simulink model "ltao_v1"  (R2022b)
settings: Solver=FixedStepDiscrete  StartTime=0.0  StopTime=0.6  FixedStep=FEM_Ts  MaxStep=FEM_Ts  RelTol=1e-2
InitFcn:
  | %
  | % Initialization callback function
  | %
  | 
  | try
  |    fprintf('\nGMT IMS version (%s)!\n',simulink_fname );
  | 
  |    % Get Simulink model directory
  |    [filepath,name,ext] = fileparts(which(bdroot));
  | 
  |    if ~strcmp(filepath,pwd)
  |       fprintf('\nChanging current directory to \n %s \n',filepath);
  |       cd(filepath);
  |    end
  | 
  |    %
  |  if(osim.bpless_wl)
  |     fprintf('Generating bumpless wind load time series\n');
  |  end
  | catch
  |    warning('Running the InitFcn from puSimulate script');
  | end
values from neighbouring files (symbols this model uses):
  asm_ssG = XiKL' * asm_ssG * XiKL    [load_ltao_e2e.m]
  Cpi_d = eye(n_Zmodes)* c2d(st.asm.fpi, Ts, c2d_opts)    [evalM2asm_modal.m]    (also in load_ltao_e2e.m = c2d(st.asm.fpi, FEM_Ts, c2d_opts))
  fao_d = c2d(st.glao.fao, st.glao.T, c2d_opts)    [evalM2asm_modal.m]    (also in load_ltao_e2e.m = c2d(st.ltao.fao, FEM_Ts, c2d_opts))
  fao_d4k = c2d(st.ltao.fao, 1/4e3, c2d_opts)    [evalM2asm_modal.m]    (also in load_ltao_e2e.m = c2d(st.ltao.fao, FEM_Ts, c2d_opts))
  FEM_Ts = 1/8e3    (= 0.000125)    [load_ltao_e2e.m]
  fes = c2d(tf((fc_es^2)*4*(pi^2),[1, 2*0.8*fc_es*2*pi, (fc_es^2)*4*(pi^2)]),     st.ltao.T,c2d_opts)    [load_ltao_e2e.m]
  flag_1stOdyn_d = tf(c2d(flag(2,1), Ts, c2d_opts))    [evalM2asm_modal.m]    (also in load_ltao_e2e.m = tf(c2d(flag(2,1),FEM_Ts,c2d_opts)))
  flag_2ndOdyn_d = tf(c2d(flag(3,1), Ts, c2d_opts))    [evalM2asm_modal.m]    (also in load_ltao_e2e.m = tf(c2d(flag(3,1),FEM_Ts,c2d_opts)))
  fpre_d = tf(c2d(st.asm.fpre, Ts, c2d_opts))    [evalM2asm_modal.m]    (also in load_ltao_e2e.m = tf(c2d(fpre,FEM_Ts,c2d_opts)))
  gtt2mnt = eye(2)/(rbm2gtt * Hk_mnt_m1m2)    [load_ltao_e2e.m]
  Hk_mnt_m1m2 = Cm1m2*pinv(Cmnt)    [load_ltao_e2e.m]
  Hpd_d = eye(n_Zmodes)* c2d(st.asm.fpd, Ts, c2d_opts)    [evalM2asm_modal.m]    (also in load_ltao_e2e.m = c2d(st.asm.fpd, FEM_Ts, 'Tustin'))
  Km1rbm_es = (KhpF2es/KhpF2m1rbm)    [load_ltao_e2e.m]
  Ks = cell(7,1)    [load_ltao_e2e.m]
  m1m2_segP_dist = [zeros(42,1); 1e-5*randn(42,1)]    [load_ltao_e2e.m]
  PG = zeros(length(om2),6)    [evalM2asm_modal.m]    (also in load_ltao_e2e.m)
  phiB = inputs2ModalF(mode_ind_vec,indDesInputs) * KinputT    [load_ltao_e2e.m]
  phiC = KoutputT * modalDisp2Outputs(indDesOutputs,mode_ind_vec)    [load_ltao_e2e.m]
  Psi_ss = KoutputT *gainMatrix(indDesOutputs,indDesInputs)* KinputT - K_ss    [load_ltao_e2e.m]
  segPTT2asmCMD = cell(7,1)    [load_ltao_e2e.m]
  Sm1m2_gtt = (Hk_mnt_m1m2*gtt2mnt) * rbm2gtt    [load_ltao_e2e.m]
  st = getcontrol_asm()    [evalM2asm_modal.m]    (also in load_ltao_e2e.m)
undefined symbols (not defined in the file or in its folder): a, az, az_ff_en, b, c, D_seg_piston, D_seg_tt, DiscIntNeverNeededParam, el, fem, gir, m1sys, m2_rbm_dist, m2pos, magnitude, mount, osim, rbm2gtt, Rm1es, Rm2es, sm, VC_modal_stiff
libraries: ims_block_library x7, simulink x2
(part 2 of 3)

== system ltao_v1/ASMmodal_Control/ASM_inner_loop_controller_S1 ==
  ASM_cmd : Inport
  ASM_FB : Inport  Port=2
  ASM Input filter : DiscreteTransferFcn  Numerator=fpre_d.num{1}  Denominator=fpre_d.den{1}  SampleTime=fpre_d.Ts
  ASM PI controller : DiscreteTransferFcn  Numerator=Cpi_d.num{1}  Denominator=Cpi_d.den{1}  SampleTime=Cpi_d.Ts
  Kb : Gain  Gain=st.asm.Kb
  Kd : Gain  Gain=st.asm.Kd
  Km : Gain  Gain=st.asm.Km
  Ks : Gain  Gain=Ks{1}  Multiplication=Matrix(K*u)
  Numerical differentiation : DiscreteTransferFcn  Numerator=Hpd_d.num{1}  Denominator=Hpd_d.den{1}  SampleTime=Hpd_d.Ts
  Sum1 : Sum  Inputs=|+-
  Sum2 : Sum
  Sum3 : Sum  Inputs=|+-
  Sum4 : Sum  Inputs=++|
  Sum5 : Sum
  m2_asm_ff_en : Gain  Gain=osim.m2_asm_ff_en
  s*fpre (DT version) : DiscreteTransferFcn  Numerator=flag_1stOdyn_d.num{1}  Denominator=flag_1stOdyn_d.den{1}  SampleTime=flag_1stOdyn_d.Ts
  s^2*fpre (DT version) : DiscreteTransferFcn  Numerator=flag_2ndOdyn_d.num{1}  Denominator=flag_2ndOdyn_d.den{1}  SampleTime=flag_2ndOdyn_d.Ts
  ASM_modalF : Outport  VectorParamsAs1DForOutWhenUnconnected=off
  Mag_modal_vel : Outport  Port=2  VectorParamsAs1DForOutWhenUnconnected=off
  wires:
  m2_asm_ff_en/1 -> Sum4/1
  s*fpre (DT version)/1 -> Kb/1
  ASM PI controller/1 -> Sum3/1
  Sum3/1 -> Sum4/2
  Km/1 -> Sum5/1
  Kb/1 -> Sum5/2
  Ks/1 -> Sum2/2
  s^2*fpre (DT version)/1 -> Km/1
  Kd/1 -> Sum3/2
  Sum5/1 -> Sum2/1
  ASM_FB/1 -> Numerical differentiation/1, Sum1/2
  ASM_cmd/1 -> s^2*fpre (DT version)/1, s*fpre (DT version)/1, ASM Input filter/1
  Sum1/1 -> ASM PI controller/1
  Sum4/1 -> ASM_modalF/1
  Sum2/1 -> m2_asm_ff_en/1
  Numerical differentiation/1 -> Mag_modal_vel/1, Kd/1
  ASM Input filter/1 -> Ks/1, Sum1/1

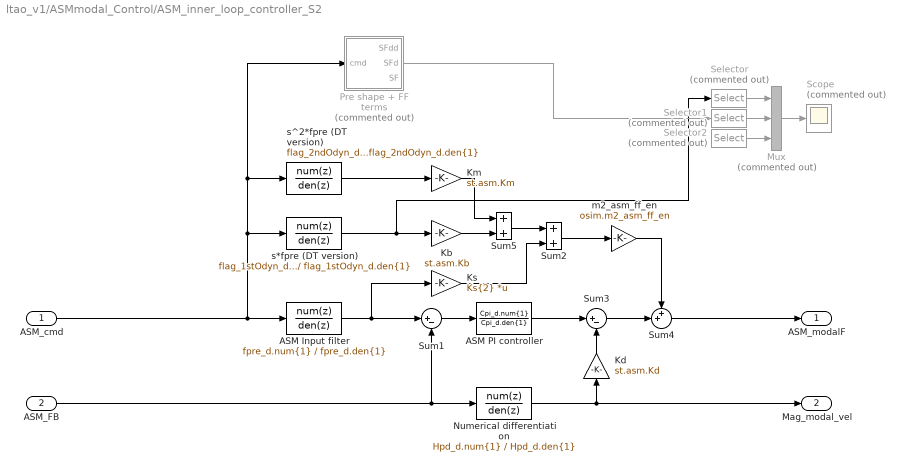
== system ltao_v1/ASMmodal_Control/ASM_inner_loop_controller_S2 ==
  ASM_cmd : Inport
  ASM_FB : Inport  Port=2
  ASM Input filter : DiscreteTransferFcn  Numerator=fpre_d.num{1}  Denominator=fpre_d.den{1}  SampleTime=fpre_d.Ts
  ASM PI controller : DiscreteTransferFcn  Numerator=Cpi_d.num{1}  Denominator=Cpi_d.den{1}  SampleTime=Cpi_d.Ts
  Kb : Gain  Gain=st.asm.Kb
  Kd : Gain  Gain=st.asm.Kd
  Km : Gain  Gain=st.asm.Km
  Ks : Gain  Gain=Ks{2}  Multiplication=Matrix(K*u)
  Mux : Mux  Commented=on  Inputs=3
  Numerical differentiation : DiscreteTransferFcn  Numerator=Hpd_d.num{1}  Denominator=Hpd_d.den{1}  SampleTime=Hpd_d.Ts
  Pre shape + FF terms : Subsystem  Commented=on
  Scope : Scope  Commented=on
  Selector : Selector  Commented=on  InputPortWidth=66  IndexOptions=Index vector (dialog)  Indices=[1 4]  OutputSizes=1
  Selector1 : Selector  Commented=on  InputPortWidth=66  IndexOptions=Index vector (dialog)  Indices=[1 4]  OutputSizes=1
  Selector2 : Selector  Commented=on  InputPortWidth=66  IndexOptions=Index vector (dialog)  Indices=[1 4]  OutputSizes=1
  Sum1 : Sum  Inputs=|+-
  Sum2 : Sum
  Sum3 : Sum  Inputs=|+-
  Sum4 : Sum  Inputs=++|
  Sum5 : Sum
  m2_asm_ff_en : Gain  Gain=osim.m2_asm_ff_en
  s*fpre (DT version) : DiscreteTransferFcn  Numerator=flag_1stOdyn_d.num{1}  Denominator=flag_1stOdyn_d.den{1}  SampleTime=flag_1stOdyn_d.Ts
  s^2*fpre (DT version) : DiscreteTransferFcn  Numerator=flag_2ndOdyn_d.num{1}  Denominator=flag_2ndOdyn_d.den{1}  SampleTime=flag_2ndOdyn_d.Ts
  ASM_modalF : Outport  VectorParamsAs1DForOutWhenUnconnected=off
  Mag_modal_vel : Outport  Port=2  VectorParamsAs1DForOutWhenUnconnected=off
  wires:
  s*fpre (DT version)/1 -> Selector/1, Kb/1
  ASM PI controller/1 -> Sum3/1
  Sum3/1 -> Sum4/2
  Km/1 -> Sum5/1
  Kb/1 -> Sum5/2
  Ks/1 -> Sum2/2
  s^2*fpre (DT version)/1 -> Km/1
  Kd/1 -> Sum3/2
  Sum5/1 -> Sum2/1
  ASM_FB/1 -> Numerical differentiation/1, Sum1/2
  ASM_cmd/1 -> Pre shape + FF terms/1(cmd), s^2*fpre (DT version)/1, s*fpre (DT version)/1, ASM Input filter/1
  Sum1/1 -> ASM PI controller/1
  Sum4/1 -> ASM_modalF/1
  Sum2/1 -> m2_asm_ff_en/1
  Numerical differentiation/1 -> Mag_modal_vel/1, Kd/1
  ASM Input filter/1 -> Ks/1, Sum1/1
  Mux/1 -> Scope/1
  Selector1/1 -> Mux/2
  Selector/1 -> Mux/1
  Selector2/1 -> Mux/3
  m2_asm_ff_en/1 -> Sum4/1
  Pre shape + FF terms/2(SFd) -> Selector1/1

== system ltao_v1/ASMmodal_Control/ASM_inner_loop_controller_S3 ==
  ASM_cmd : Inport
  ASM_FB : Inport  Port=2
  ASM Input filter : DiscreteTransferFcn  Numerator=fpre_d.num{1}  Denominator=fpre_d.den{1}  SampleTime=fpre_d.Ts
  ASM PI controller : DiscreteTransferFcn  Numerator=Cpi_d.num{1}  Denominator=Cpi_d.den{1}  SampleTime=Cpi_d.Ts
  Kb : Gain  Gain=st.asm.Kb
  Kd : Gain  Gain=st.asm.Kd
  Km : Gain  Gain=st.asm.Km
  Ks : Gain  Gain=Ks{3}  Multiplication=Matrix(K*u)
  Numerical differentiation : DiscreteTransferFcn  Numerator=Hpd_d.num{1}  Denominator=Hpd_d.den{1}  SampleTime=Hpd_d.Ts
  Sum1 : Sum  Inputs=|+-
  Sum2 : Sum
  Sum3 : Sum  Inputs=|+-
  Sum4 : Sum  Inputs=++|
  Sum5 : Sum
  m2_asm_ff_en : Gain  Gain=osim.m2_asm_ff_en
  s*fpre (DT version) : DiscreteTransferFcn  Numerator=flag_1stOdyn_d.num{1}  Denominator=flag_1stOdyn_d.den{1}  SampleTime=flag_1stOdyn_d.Ts
  s^2*fpre (DT version) : DiscreteTransferFcn  Numerator=flag_2ndOdyn_d.num{1}  Denominator=flag_2ndOdyn_d.den{1}  SampleTime=flag_2ndOdyn_d.Ts
  ASM_modalF : Outport  VectorParamsAs1DForOutWhenUnconnected=off
  Mag_modal_vel : Outport  Port=2  VectorParamsAs1DForOutWhenUnconnected=off
  wires:
  m2_asm_ff_en/1 -> Sum4/1
  s*fpre (DT version)/1 -> Kb/1
  ASM PI controller/1 -> Sum3/1
  Sum3/1 -> Sum4/2
  Km/1 -> Sum5/1
  Kb/1 -> Sum5/2
  Ks/1 -> Sum2/2
  s^2*fpre (DT version)/1 -> Km/1
  Kd/1 -> Sum3/2
  Sum5/1 -> Sum2/1
  ASM_FB/1 -> Numerical differentiation/1, Sum1/2
  ASM_cmd/1 -> s^2*fpre (DT version)/1, s*fpre (DT version)/1, ASM Input filter/1
  Sum1/1 -> ASM PI controller/1
  Sum4/1 -> ASM_modalF/1
  Sum2/1 -> m2_asm_ff_en/1
  Numerical differentiation/1 -> Mag_modal_vel/1, Kd/1
  ASM Input filter/1 -> Ks/1, Sum1/1

== system ltao_v1/ASMmodal_Control/ASM_inner_loop_controller_S4 ==
  ASM_cmd : Inport
  ASM_FB : Inport  Port=2
  ASM Input filter : DiscreteTransferFcn  Numerator=fpre_d.num{1}  Denominator=fpre_d.den{1}  SampleTime=fpre_d.Ts
  ASM PI controller : DiscreteTransferFcn  Numerator=Cpi_d.num{1}  Denominator=Cpi_d.den{1}  SampleTime=Cpi_d.Ts
  Kb : Gain  Gain=st.asm.Kb
  Kd : Gain  Gain=st.asm.Kd
  Km : Gain  Gain=st.asm.Km
  Ks : Gain  Gain=Ks{4}  Multiplication=Matrix(K*u)
  Numerical differentiation : DiscreteTransferFcn  Numerator=Hpd_d.num{1}  Denominator=Hpd_d.den{1}  SampleTime=Hpd_d.Ts
  Sum1 : Sum  Inputs=|+-
  Sum2 : Sum
  Sum3 : Sum  Inputs=|+-
  Sum4 : Sum  Inputs=++|
  Sum5 : Sum
  m2_asm_ff_en : Gain  Gain=osim.m2_asm_ff_en
  s*fpre (DT version) : DiscreteTransferFcn  Numerator=flag_1stOdyn_d.num{1}  Denominator=flag_1stOdyn_d.den{1}  SampleTime=flag_1stOdyn_d.Ts
  s^2*fpre (DT version) : DiscreteTransferFcn  Numerator=flag_2ndOdyn_d.num{1}  Denominator=flag_2ndOdyn_d.den{1}  SampleTime=flag_2ndOdyn_d.Ts
  ASM_modalF : Outport  VectorParamsAs1DForOutWhenUnconnected=off
  Mag_modal_vel : Outport  Port=2  VectorParamsAs1DForOutWhenUnconnected=off
  wires:
  m2_asm_ff_en/1 -> Sum4/1
  s*fpre (DT version)/1 -> Kb/1
  ASM PI controller/1 -> Sum3/1
  Sum3/1 -> Sum4/2
  Km/1 -> Sum5/1
  Kb/1 -> Sum5/2
  Ks/1 -> Sum2/2
  s^2*fpre (DT version)/1 -> Km/1
  Kd/1 -> Sum3/2
  Sum5/1 -> Sum2/1
  ASM_FB/1 -> Numerical differentiation/1, Sum1/2
  ASM_cmd/1 -> s^2*fpre (DT version)/1, s*fpre (DT version)/1, ASM Input filter/1
  Sum1/1 -> ASM PI controller/1
  Sum4/1 -> ASM_modalF/1
  Sum2/1 -> m2_asm_ff_en/1
  Numerical differentiation/1 -> Mag_modal_vel/1, Kd/1
  ASM Input filter/1 -> Ks/1, Sum1/1

== system ltao_v1/ASMmodal_Control/ASM_inner_loop_controller_S5 ==
  ASM_cmd : Inport
  ASM_FB : Inport  Port=2
  ASM Input filter : DiscreteTransferFcn  Numerator=fpre_d.num{1}  Denominator=fpre_d.den{1}  SampleTime=fpre_d.Ts
  ASM PI controller : DiscreteTransferFcn  Numerator=Cpi_d.num{1}  Denominator=Cpi_d.den{1}  SampleTime=Cpi_d.Ts
  Kb : Gain  Gain=st.asm.Kb
  Kd : Gain  Gain=st.asm.Kd
  Km : Gain  Gain=st.asm.Km
  Ks : Gain  Gain=Ks{5}  Multiplication=Matrix(K*u)
  Numerical differentiation : DiscreteTransferFcn  Numerator=Hpd_d.num{1}  Denominator=Hpd_d.den{1}  SampleTime=Hpd_d.Ts
  Sum1 : Sum  Inputs=|+-
  Sum2 : Sum
  Sum3 : Sum  Inputs=|+-
  Sum4 : Sum  Inputs=++|
  Sum5 : Sum
  m2_asm_ff_en : Gain  Gain=osim.m2_asm_ff_en
  s*fpre (DT version) : DiscreteTransferFcn  Numerator=flag_1stOdyn_d.num{1}  Denominator=flag_1stOdyn_d.den{1}  SampleTime=flag_1stOdyn_d.Ts
  s^2*fpre (DT version) : DiscreteTransferFcn  Numerator=flag_2ndOdyn_d.num{1}  Denominator=flag_2ndOdyn_d.den{1}  SampleTime=flag_2ndOdyn_d.Ts
  ASM_modalF : Outport  VectorParamsAs1DForOutWhenUnconnected=off
  Mag_modal_vel : Outport  Port=2  VectorParamsAs1DForOutWhenUnconnected=off
  wires:
  m2_asm_ff_en/1 -> Sum4/1
  s*fpre (DT version)/1 -> Kb/1
  ASM PI controller/1 -> Sum3/1
  Sum3/1 -> Sum4/2
  Km/1 -> Sum5/1
  Kb/1 -> Sum5/2
  Ks/1 -> Sum2/2
  s^2*fpre (DT version)/1 -> Km/1
  Kd/1 -> Sum3/2
  Sum5/1 -> Sum2/1
  ASM_FB/1 -> Numerical differentiation/1, Sum1/2
  ASM_cmd/1 -> s^2*fpre (DT version)/1, s*fpre (DT version)/1, ASM Input filter/1
  Sum1/1 -> ASM PI controller/1
  Sum4/1 -> ASM_modalF/1
  Sum2/1 -> m2_asm_ff_en/1
  Numerical differentiation/1 -> Mag_modal_vel/1, Kd/1
  ASM Input filter/1 -> Ks/1, Sum1/1

== system ltao_v1/ASMmodal_Control/ASM_inner_loop_controller_S6 ==
  ASM_cmd : Inport
  ASM_FB : Inport  Port=2
  ASM Input filter : DiscreteTransferFcn  Numerator=fpre_d.num{1}  Denominator=fpre_d.den{1}  SampleTime=fpre_d.Ts
  ASM PI controller : DiscreteTransferFcn  Numerator=Cpi_d.num{1}  Denominator=Cpi_d.den{1}  SampleTime=Cpi_d.Ts
  Kb : Gain  Gain=st.asm.Kb
  Kd : Gain  Gain=st.asm.Kd
  Km : Gain  Gain=st.asm.Km
  Ks : Gain  Gain=Ks{6}  Multiplication=Matrix(K*u)
  Numerical differentiation : DiscreteTransferFcn  Numerator=Hpd_d.num{1}  Denominator=Hpd_d.den{1}  SampleTime=Hpd_d.Ts
  Sum1 : Sum  Inputs=|+-
  Sum2 : Sum
  Sum3 : Sum  Inputs=|+-
  Sum4 : Sum  Inputs=++|
  Sum5 : Sum
  m2_asm_ff_en : Gain  Gain=osim.m2_asm_ff_en
  s*fpre (DT version) : DiscreteTransferFcn  Numerator=flag_1stOdyn_d.num{1}  Denominator=flag_1stOdyn_d.den{1}  SampleTime=flag_1stOdyn_d.Ts
  s^2*fpre (DT version) : DiscreteTransferFcn  Numerator=flag_2ndOdyn_d.num{1}  Denominator=flag_2ndOdyn_d.den{1}  SampleTime=flag_2ndOdyn_d.Ts
  ASM_modalF : Outport  VectorParamsAs1DForOutWhenUnconnected=off
  Mag_modal_vel : Outport  Port=2  VectorParamsAs1DForOutWhenUnconnected=off
  wires:
  m2_asm_ff_en/1 -> Sum4/1
  s*fpre (DT version)/1 -> Kb/1
  ASM PI controller/1 -> Sum3/1
  Sum3/1 -> Sum4/2
  Km/1 -> Sum5/1
  Kb/1 -> Sum5/2
  Ks/1 -> Sum2/2
  s^2*fpre (DT version)/1 -> Km/1
  Kd/1 -> Sum3/2
  Sum5/1 -> Sum2/1
  ASM_FB/1 -> Numerical differentiation/1, Sum1/2
  ASM_cmd/1 -> s^2*fpre (DT version)/1, s*fpre (DT version)/1, ASM Input filter/1
  Sum1/1 -> ASM PI controller/1
  Sum4/1 -> ASM_modalF/1
  Sum2/1 -> m2_asm_ff_en/1
  Numerical differentiation/1 -> Mag_modal_vel/1, Kd/1
  ASM Input filter/1 -> Ks/1, Sum1/1

== system ltao_v1/ASMmodal_Control/ASM_inner_loop_controller_S7 ==
  ASM_cmd : Inport
  ASM_FB : Inport  Port=2
  ASM Input filter : DiscreteTransferFcn  Numerator=fpre_d.num{1}  Denominator=fpre_d.den{1}  SampleTime=fpre_d.Ts
  ASM PI controller : DiscreteTransferFcn  Numerator=Cpi_d.num{1}  Denominator=Cpi_d.den{1}  SampleTime=Cpi_d.Ts
  Kb : Gain  Gain=st.asm.Kb
  Kd : Gain  Gain=st.asm.Kd
  Km : Gain  Gain=st.asm.Km
  Ks : Gain  Gain=Ks{7}  Multiplication=Matrix(K*u)
  Numerical differentiation : DiscreteTransferFcn  Numerator=Hpd_d.num{1}  Denominator=Hpd_d.den{1}  SampleTime=Hpd_d.Ts
  Sum1 : Sum  Inputs=|+-
  Sum2 : Sum
  Sum3 : Sum  Inputs=|+-
  Sum4 : Sum  Inputs=++|
  Sum5 : Sum
  m2_asm_ff_en : Gain  Gain=osim.m2_asm_ff_en
  s*fpre (DT version) : DiscreteTransferFcn  Numerator=flag_1stOdyn_d.num{1}  Denominator=flag_1stOdyn_d.den{1}  SampleTime=flag_1stOdyn_d.Ts
  s^2*fpre (DT version) : DiscreteTransferFcn  Numerator=flag_2ndOdyn_d.num{1}  Denominator=flag_2ndOdyn_d.den{1}  SampleTime=flag_2ndOdyn_d.Ts
  ASM_modalF : Outport  VectorParamsAs1DForOutWhenUnconnected=off
  Mag_modal_vel : Outport  Port=2  VectorParamsAs1DForOutWhenUnconnected=off
  wires:
  m2_asm_ff_en/1 -> Sum4/1
  s*fpre (DT version)/1 -> Kb/1
  ASM PI controller/1 -> Sum3/1
  Sum3/1 -> Sum4/2
  Km/1 -> Sum5/1
  Kb/1 -> Sum5/2
  Ks/1 -> Sum2/2
  s^2*fpre (DT version)/1 -> Km/1
  Kd/1 -> Sum3/2
  Sum5/1 -> Sum2/1
  ASM_FB/1 -> Numerical differentiation/1, Sum1/2
  ASM_cmd/1 -> s^2*fpre (DT version)/1, s*fpre (DT version)/1, ASM Input filter/1
  Sum1/1 -> ASM PI controller/1
  Sum4/1 -> ASM_modalF/1
  Sum2/1 -> m2_asm_ff_en/1
  Numerical differentiation/1 -> Mag_modal_vel/1, Kd/1
  ASM Input filter/1 -> Ks/1, Sum1/1

== system ltao_v1/LTWS Controller/segPTT2asmCMD ==
  segTTP : Inport
  Mux : Mux  Inputs=7
  PTT2ASM_S1 : Gain  Gain=segPTT2asmCMD{1}  Multiplication=Matrix(K*u)
  PTT2ASM_S2 : Gain  Gain=segPTT2asmCMD{2}  Multiplication=Matrix(K*u)
  PTT2ASM_S3 : Gain  Gain=segPTT2asmCMD{3}  Multiplication=Matrix(K*u)
  PTT2ASM_S4 : Gain  Gain=segPTT2asmCMD{4}  Multiplication=Matrix(K*u)
  PTT2ASM_S5 : Gain  Gain=segPTT2asmCMD{5}  Multiplication=Matrix(K*u)
  PTT2ASM_S6 : Gain  Gain=segPTT2asmCMD{6}  Multiplication=Matrix(K*u)
  PTT2ASM_S7 : Gain  Gain=segPTT2asmCMD{7}  Multiplication=Matrix(K*u)
  Selector_S1 : Selector  InputPortWidth=21  IndexOptions=Index vector (dialog)  Indices=1:7:21  OutputSizes=1
  Selector_S2 : Selector  InputPortWidth=21  IndexOptions=Index vector (dialog)  Indices=2:7:21  OutputSizes=1
  Selector_S3 : Selector  InputPortWidth=21  IndexOptions=Index vector (dialog)  Indices=3:7:21  OutputSizes=1
  Selector_S4 : Selector  InputPortWidth=21  IndexOptions=Index vector (dialog)  Indices=4:7:21  OutputSizes=1
  Selector_S5 : Selector  InputPortWidth=21  IndexOptions=Index vector (dialog)  Indices=5:7:21  OutputSizes=1
  Selector_S6 : Selector  InputPortWidth=21  IndexOptions=Index vector (dialog)  Indices=6:7:21  OutputSizes=1
  Selector_S7 : Selector  InputPortWidth=21  IndexOptions=Index vector (dialog)  Indices=7:7:21  OutputSizes=1
  ASM_KL012_CMD : Outport
  wires:
  Mux/1 -> ASM_KL012_CMD/1
  PTT2ASM_S7/1 -> Mux/7
  PTT2ASM_S6/1 -> Mux/6
  PTT2ASM_S5/1 -> Mux/5
  PTT2ASM_S3/1 -> Mux/3
  PTT2ASM_S4/1 -> Mux/4
  PTT2ASM_S2/1 -> Mux/2
  Selector_S4/1 -> PTT2ASM_S4/1
  PTT2ASM_S1/1 -> Mux/1
  Selector_S7/1 -> PTT2ASM_S7/1
  Selector_S6/1 -> PTT2ASM_S6/1
  Selector_S3/1 -> PTT2ASM_S3/1
  Selector_S2/1 -> PTT2ASM_S2/1
  Selector_S1/1 -> PTT2ASM_S1/1
  Selector_S5/1 -> PTT2ASM_S5/1
  segTTP/1 -> Selector_S7/1, Selector_S6/1, Selector_S5/1, Selector_S4/1, Selector_S3/1, Selector_S2/1, Selector_S1/1

== system ltao_v1/M1 ES FF/segPTT2asmCMD ==
  segTTP : Inport
  Mux : Mux  Inputs=7
  PTT2ASM_S1 : Gain  Gain=segPTT2asmCMD{1}  Multiplication=Matrix(K*u)
  PTT2ASM_S2 : Gain  Gain=segPTT2asmCMD{2}  Multiplication=Matrix(K*u)
  PTT2ASM_S3 : Gain  Gain=segPTT2asmCMD{3}  Multiplication=Matrix(K*u)
  PTT2ASM_S4 : Gain  Gain=segPTT2asmCMD{4}  Multiplication=Matrix(K*u)
  PTT2ASM_S5 : Gain  Gain=segPTT2asmCMD{5}  Multiplication=Matrix(K*u)
  PTT2ASM_S6 : Gain  Gain=segPTT2asmCMD{6}  Multiplication=Matrix(K*u)
  PTT2ASM_S7 : Gain  Gain=segPTT2asmCMD{7}  Multiplication=Matrix(K*u)
  Selector_S1 : Selector  InputPortWidth=21  IndexOptions=Index vector (dialog)  Indices=1:7:21  OutputSizes=1
  Selector_S2 : Selector  InputPortWidth=21  IndexOptions=Index vector (dialog)  Indices=2:7:21  OutputSizes=1
  Selector_S3 : Selector  InputPortWidth=21  IndexOptions=Index vector (dialog)  Indices=3:7:21  OutputSizes=1
  Selector_S4 : Selector  InputPortWidth=21  IndexOptions=Index vector (dialog)  Indices=4:7:21  OutputSizes=1
  Selector_S5 : Selector  InputPortWidth=21  IndexOptions=Index vector (dialog)  Indices=5:7:21  OutputSizes=1
  Selector_S6 : Selector  InputPortWidth=21  IndexOptions=Index vector (dialog)  Indices=6:7:21  OutputSizes=1
  Selector_S7 : Selector  InputPortWidth=21  IndexOptions=Index vector (dialog)  Indices=7:7:21  OutputSizes=1
  ASM_KL012_CMD : Outport
  wires:
  Mux/1 -> ASM_KL012_CMD/1
  PTT2ASM_S7/1 -> Mux/7
  PTT2ASM_S6/1 -> Mux/6
  PTT2ASM_S5/1 -> Mux/5
  PTT2ASM_S3/1 -> Mux/3
  PTT2ASM_S4/1 -> Mux/4
  PTT2ASM_S2/1 -> Mux/2
  Selector_S4/1 -> PTT2ASM_S4/1
  PTT2ASM_S1/1 -> Mux/1
  Selector_S7/1 -> PTT2ASM_S7/1
  Selector_S6/1 -> PTT2ASM_S6/1
  Selector_S3/1 -> PTT2ASM_S3/1
  Selector_S2/1 -> PTT2ASM_S2/1
  Selector_S1/1 -> PTT2ASM_S1/1
  Selector_S5/1 -> PTT2ASM_S5/1
  segTTP/1 -> Selector_S7/1, Selector_S6/1, Selector_S5/1, Selector_S4/1, Selector_S3/1, Selector_S2/1, Selector_S1/1

== system ltao_v1/M1_HP_loadcells/M1S1 Loadcell ==
  note: HP Forces
  note: HP Relative
      | Displacements
  HP_F_cmd : Inport
  HP_D_cell : Inport  Port=2
  HP_D_face : Inport  Port=3
  HpK : Gain  Gain=m1sys{1}.HPstiff
  Sum1 : Sum  Inputs=-+|
  Sum9 : Sum  Inputs=-+|
  HP_F_meas : Outport  VectorParamsAs1DForOutWhenUnconnected=off
  wires:
  HP_D_cell/1 -> Sum9/1
  HP_D_face/1 -> Sum9/2
  Sum9/1 -> HpK/1
  HpK/1 -> Sum1/2
  Sum1/1 -> HP_F_meas/1
  HP_F_cmd/1 -> Sum1/1

== system ltao_v1/M1_HP_loadcells/M1S2 Loadcell ==
  note: HP Relative
      | Displacements
  note: HP Forces
  HP_F_cmd : Inport
  HP_D_cell : Inport  Port=2
  HP_D_face : Inport  Port=3
  HpK : Gain  Gain=m1sys{2}.HPstiff
  Sum1 : Sum  Inputs=-+|
  Sum9 : Sum  Inputs=-+|
  HP_F_meas : Outport  VectorParamsAs1DForOutWhenUnconnected=off
  wires:
  HP_D_face/1 -> Sum9/2
  HP_D_cell/1 -> Sum9/1
  HP_F_cmd/1 -> Sum1/1
  HpK/1 -> Sum1/2
  Sum1/1 -> HP_F_meas/1
  Sum9/1 -> HpK/1

== system ltao_v1/M1_HP_loadcells/M1S3 Loadcell ==
  note: HP Relative
      | Displacements
  note: HP Forces
  HP_F_cmd : Inport
  HP_D_cell : Inport  Port=2
  HP_D_face : Inport  Port=3
  HpK : Gain  Gain=m1sys{3}.HPstiff
  Sum1 : Sum  Inputs=-+|
  Sum9 : Sum  Inputs=-+|
  HP_F_meas : Outport  VectorParamsAs1DForOutWhenUnconnected=off
  wires:
  HP_D_face/1 -> Sum9/2
  HP_D_cell/1 -> Sum9/1
  HP_F_cmd/1 -> Sum1/1
  HpK/1 -> Sum1/2
  Sum1/1 -> HP_F_meas/1
  Sum9/1 -> HpK/1

== system ltao_v1/M1_HP_loadcells/M1S4 Loadcell ==
  note: HP Relative
      | Displacements
  note: HP Forces
  HP_F_cmd : Inport
  HP_D_cell : Inport  Port=2
  HP_D_face : Inport  Port=3
  HpK : Gain  Gain=m1sys{4}.HPstiff
  Sum1 : Sum  Inputs=-+|
  Sum9 : Sum  Inputs=-+|
  HP_F_meas : Outport  VectorParamsAs1DForOutWhenUnconnected=off
  wires:
  HP_D_face/1 -> Sum9/2
  HP_D_cell/1 -> Sum9/1
  HP_F_cmd/1 -> Sum1/1
  HpK/1 -> Sum1/2
  Sum1/1 -> HP_F_meas/1
  Sum9/1 -> HpK/1

== system ltao_v1/M1_HP_loadcells/M1S5 Loadcell ==
  note: HP Relative
      | Displacements
  note: HP Forces
  HP_F_cmd : Inport
  HP_D_cell : Inport  Port=2
  HP_D_face : Inport  Port=3
  HpK : Gain  Gain=m1sys{5}.HPstiff
  Sum1 : Sum  Inputs=-+|
  Sum9 : Sum  Inputs=-+|
  HP_F_meas : Outport  VectorParamsAs1DForOutWhenUnconnected=off
  wires:
  HP_D_face/1 -> Sum9/2
  HP_D_cell/1 -> Sum9/1
  HP_F_cmd/1 -> Sum1/1
  HpK/1 -> Sum1/2
  Sum1/1 -> HP_F_meas/1
  Sum9/1 -> HpK/1

== system ltao_v1/M1_HP_loadcells/M1S6 Loadcell ==
  note: HP Relative
      | Displacements
  note: HP Forces
  HP_F_cmd : Inport
  HP_D_cell : Inport  Port=2
  HP_D_face : Inport  Port=3
  HpK : Gain  Gain=m1sys{6}.HPstiff
  Sum1 : Sum  Inputs=-+|
  Sum9 : Sum  Inputs=-+|
  HP_F_meas : Outport  VectorParamsAs1DForOutWhenUnconnected=off
  wires:
  HP_D_face/1 -> Sum9/2
  HP_D_cell/1 -> Sum9/1
  HP_F_cmd/1 -> Sum1/1
  HpK/1 -> Sum1/2
  Sum1/1 -> HP_F_meas/1
  Sum9/1 -> HpK/1

== system ltao_v1/M1_HP_loadcells/M1S7 Control ==
  note: HP Relative
      | Displacements
  note: HP Forces
  HP_F_cmd : Inport
  HP_D_cell : Inport  Port=2
  HP_D_face : Inport  Port=3
  HpK : Gain  Gain=m1sys{7}.HPstiff
  Sum1 : Sum  Inputs=-+|
  Sum9 : Sum  Inputs=-+|
  HP_F_meas : Outport  VectorParamsAs1DForOutWhenUnconnected=off
  wires:
  HP_D_face/1 -> Sum9/2
  HP_D_cell/1 -> Sum9/1
  HP_F_cmd/1 -> Sum1/1
  HpK/1 -> Sum1/2
  Sum1/1 -> HP_F_meas/1
  Sum9/1 -> HpK/1

== system ltao_v1/M2 ES FF/segPTT2asmCMD ==
  segTTP : Inport
  Mux : Mux  Inputs=7
  PTT2ASM_S1 : Gain  Gain=segPTT2asmCMD{1}  Multiplication=Matrix(K*u)
  PTT2ASM_S2 : Gain  Gain=segPTT2asmCMD{2}  Multiplication=Matrix(K*u)
  PTT2ASM_S3 : Gain  Gain=segPTT2asmCMD{3}  Multiplication=Matrix(K*u)
  PTT2ASM_S4 : Gain  Gain=segPTT2asmCMD{4}  Multiplication=Matrix(K*u)
  PTT2ASM_S5 : Gain  Gain=segPTT2asmCMD{5}  Multiplication=Matrix(K*u)
  PTT2ASM_S6 : Gain  Gain=segPTT2asmCMD{6}  Multiplication=Matrix(K*u)
  PTT2ASM_S7 : Gain  Gain=segPTT2asmCMD{7}  Multiplication=Matrix(K*u)
  Selector_S1 : Selector  InputPortWidth=21  IndexOptions=Index vector (dialog)  Indices=1:7:21  OutputSizes=1
  Selector_S2 : Selector  InputPortWidth=21  IndexOptions=Index vector (dialog)  Indices=2:7:21  OutputSizes=1
  Selector_S3 : Selector  InputPortWidth=21  IndexOptions=Index vector (dialog)  Indices=3:7:21  OutputSizes=1
  Selector_S4 : Selector  InputPortWidth=21  IndexOptions=Index vector (dialog)  Indices=4:7:21  OutputSizes=1
  Selector_S5 : Selector  InputPortWidth=21  IndexOptions=Index vector (dialog)  Indices=5:7:21  OutputSizes=1
  Selector_S6 : Selector  InputPortWidth=21  IndexOptions=Index vector (dialog)  Indices=6:7:21  OutputSizes=1
  Selector_S7 : Selector  InputPortWidth=21  IndexOptions=Index vector (dialog)  Indices=7:7:21  OutputSizes=1
  ASM_KL012_CMD : Outport
  wires:
  Mux/1 -> ASM_KL012_CMD/1
  PTT2ASM_S7/1 -> Mux/7
  PTT2ASM_S6/1 -> Mux/6
  PTT2ASM_S5/1 -> Mux/5
  PTT2ASM_S3/1 -> Mux/3
  PTT2ASM_S4/1 -> Mux/4
  PTT2ASM_S2/1 -> Mux/2
  Selector_S4/1 -> PTT2ASM_S4/1
  PTT2ASM_S1/1 -> Mux/1
  Selector_S7/1 -> PTT2ASM_S7/1
  Selector_S6/1 -> PTT2ASM_S6/1
  Selector_S3/1 -> PTT2ASM_S3/1
  Selector_S2/1 -> PTT2ASM_S2/1
  Selector_S1/1 -> PTT2ASM_S1/1
  Selector_S5/1 -> PTT2ASM_S5/1
  segTTP/1 -> Selector_S7/1, Selector_S6/1, Selector_S5/1, Selector_S4/1, Selector_S3/1, Selector_S2/1, Selector_S1/1

== system ltao_v1/Mount_Control/DT_siso_SS ==
  In1 : Inport
  A : Gain  Gain=a  Multiplication=Matrix(K*u) (u vector)
  Add : Sum
  B : Gain  Gain=b
  C : Gain  Gain=c
  Unit Delay : UnitDelay  SampleTime=-1  HasFrameUpgradeWarning=on
  Out1 : Outport
  wires:
  In1/1 -> B/1
  C/1 -> Out1/1
  B/1 -> Add/1
  Add/1 -> Unit Delay/1
  A/1 -> Add/2
  Unit Delay/1 -> A/1, C/1

== system ltao_v1/Mount_Drv_PDR2021_linear/AZ DT Lugre Fr model ==
  vel : Inport
  Enable : EnablePort
  Constant : Constant  Value=frParStruct.iIsSig01Active
  Discrete-Time Integrator : DiscreteIntegrator  SampleTime=-1  ICPrevOutput=DiscIntNeverNeededParam  ICPrevScaledInput=DiscIntNeverNeededParam
  Sum : Sum  Inputs=+++
  g(v) : Subsystem
  sigma_0 : Gain  Gain=frParStruct.sigm0
  sigma_1 : Gain  Gain=frParStruct.sigm1
  sigma_v : Gain  Gain=frParStruct.sigmv
  v2z : Subsystem
  FrTorque : Outport  VectorParamsAs1DForOutWhenUnconnected=off
  wires:
  Discrete-Time Integrator/1 -> sigma_0/1, v2z/3(z)
  g(v)/1(g) -> v2z/2(g(v))
  sigma_v/1 -> Sum/3  "Viscose Friction"
  v2z/1(dz) -> Discrete-Time Integrator/1, sigma_1/1
  sigma_1/1 -> Sum/1
  sigma_0/1 -> Sum/2
  Sum/1 -> FrTorque/1
  vel/1 -> v2z/1(v), g(v)/1(v), sigma_v/1
  Constant/1 -> g(v)/Enable, v2z/Enable

== system ltao_v1/Mount_Drv_PDR2021_linear/EL DT Lugre Fr model ==
  vel : Inport
  Enable : EnablePort
  Constant : Constant  Value=frParStruct.iIsSig01Active
  Discrete-Time Integrator : DiscreteIntegrator  SampleTime=-1  ICPrevOutput=DiscIntNeverNeededParam  ICPrevScaledInput=DiscIntNeverNeededParam
  Sum : Sum  Inputs=+++
  To Workspace : ToWorkspace  VariableName=el_Ve  SampleTime=-1
  To Workspace1 : ToWorkspace  VariableName=el_To  SampleTime=-1
  g(v) : Subsystem
  sigma_0 : Gain  Gain=frParStruct.sigm0
  sigma_1 : Gain  Gain=frParStruct.sigm1
  sigma_v : Gain  Gain=frParStruct.sigmv
  v2z : Subsystem
  FrTorque : Outport  VectorParamsAs1DForOutWhenUnconnected=off
  wires:
  sigma_v/1 -> Sum/3  "Viscose Friction"
  vel/1 -> v2z/1(v), g(v)/1(v), To Workspace/1, sigma_v/1
  Constant/1 -> g(v)/Enable, v2z/Enable
  sigma_0/1 -> Sum/2
  g(v)/1(g) -> v2z/2(g(v))
  sigma_1/1 -> Sum/1
  Discrete-Time Integrator/1 -> sigma_0/1, v2z/3(z)
  v2z/1(dz) -> Discrete-Time Integrator/1, sigma_1/1
  Sum/1 -> To Workspace1/1, FrTorque/1

== system ltao_v1/Mount_Drv_PDR2021_linear/GIR DT Lugre Fr model ==
  vel : Inport
  Enable : EnablePort
  Discrete-Time Integrator : DiscreteIntegrator  SampleTime=-1  ICPrevOutput=DiscIntNeverNeededParam  ICPrevScaledInput=DiscIntNeverNeededParam
  Gain : Gain  Gain=frParStruct.iIsSig01Active
  Scope : Scope
  Sum : Sum  Inputs=+++
  To Workspace : ToWorkspace  VariableName=gir_Ve  SampleTime=-1
  To Workspace1 : ToWorkspace  VariableName=gir_To  SampleTime=-1
  g(v) : Subsystem
  sigma_0 : Gain  Gain=frParStruct.sigm0
  sigma_1 : Gain  Gain=frParStruct.sigm1
  sigma_v : Gain  Gain=frParStruct.sigmv
  v2z : Subsystem
  FrTorque : Outport  VectorParamsAs1DForOutWhenUnconnected=off
  wires:
  sigma_v/1 -> Sum/3  "Viscose Friction"
  vel/1 -> Gain/1, To Workspace/1, sigma_v/1
  sigma_0/1 -> Sum/2
  g(v)/1(g) -> v2z/2(g(v))
  Discrete-Time Integrator/1 -> sigma_0/1, v2z/3(z)
  v2z/1(dz) -> Discrete-Time Integrator/1, Scope/1, sigma_1/1
  Sum/1 -> To Workspace1/1, FrTorque/1
  sigma_1/1 -> Sum/1
  Gain/1 -> v2z/1(v), g(v)/1(v)

== system ltao_v1/Mount_Drv_PDR2021_linear/Parasitic torques model  ==
  Az_pos_drv : Inport
  El_pos_drv : Inport  Port=2
  Gir_pos_drv : Inport  Port=3
  Az_drv_to : Inport  Port=4
  El_drv_to : Inport  Port=5
  Gir_drv_to : Inport  Port=6
  AZ_Parasitic_Torque : Subsystem  mask{ParasiticModelStruc=mount.az.ParasiticTo}
      mask prompts: ParasiticModelStruc "Parasitic Torque Model Parameters Structure"
  EL_Parasitic_Torque : Subsystem  mask{ParasiticModelStruc=mount.el.ParasiticTo}
      mask prompts: ParasiticModelStruc "Parasitic Torque Model Parameters Structure"
  GIR_Parasitic_Torque : Subsystem  mask{ParasiticModelStruc=mount.gir.ParasiticTo, T_pretension=mount.gir.T_pretension}
      mask prompts: ParasiticModelStruc "Parasitic Torque Model Parameters Structure"; T_pretension "Pretension torque"
  Mux1 : Mux  Commented=on  Inputs=2
  Mux2 : Mux  Commented=on  Inputs=2
  Mux6 : Mux  Commented=on  Inputs=2
  ParTo_Scope : Scope  Commented=on  NumInputPorts=3
  Subsystem : Subsystem  Commented=on
  Az_Par_To : Outport  VectorParamsAs1DForOutWhenUnconnected=off
  El_Par_To : Outport  Port=2  VectorParamsAs1DForOutWhenUnconnected=off
  Gir_Par_To : Outport  Port=3  VectorParamsAs1DForOutWhenUnconnected=off
  wires:
  Az_drv_to/1 -> Subsystem/2(Az To), AZ_Parasitic_Torque/2(Drive_Torque)
  Gir_drv_to/1 -> Subsystem/6(Gir To), GIR_Parasitic_Torque/2(Drive_Torque)
  GIR_Parasitic_Torque/1(Parasitic_Torque) -> Gir_Par_To/1, Mux6/1
  Gir_pos_drv/1 -> Subsystem/5(Gir Pos), GIR_Parasitic_Torque/1(Drive_Pos)
  El_drv_to/1 -> Subsystem/4(El To), EL_Parasitic_Torque/2(Drive_Torque)
  Az_pos_drv/1 -> Subsystem/1(Az Pos), AZ_Parasitic_Torque/1(Drive_Pos)
  El_pos_drv/1 -> Subsystem/3(El Pos), EL_Parasitic_Torque/1(Drive_Pos)
  AZ_Parasitic_Torque/1(Parasitic_Torque) -> Mux2/1, Az_Par_To/1
  EL_Parasitic_Torque/1(Parasitic_Torque) -> El_Par_To/1, Mux1/1
  Mux2/1 -> ParTo_Scope/1
  Mux1/1 -> ParTo_Scope/2
  Mux6/1 -> ParTo_Scope/3
  Subsystem/1(Out1) -> Mux2/2
  Subsystem/2(Out2) -> Mux1/2
  Subsystem/3(Out3) -> Mux6/2

== system ltao_v1/Segment TT/LOS Selector ==
  FP : Inport
  Selector : Selector  InputPortWidth=14  IndexOptions=Index vector (dialog)  Indices=[1:7]  OutputSizes=1
  Selector1 : Selector  InputPortWidth=14  IndexOptions=Index vector (dialog)  Indices=[8:14]  OutputSizes=1
  LOS X : Outport  VectorParamsAs1DForOutWhenUnconnected=off
  LOS Y : Outport  Port=2  VectorParamsAs1DForOutWhenUnconnected=off
  wires:
  FP/1 -> Selector/1, Selector1/1
  Selector1/1 -> LOS Y/1
  Selector/1 -> LOS X/1

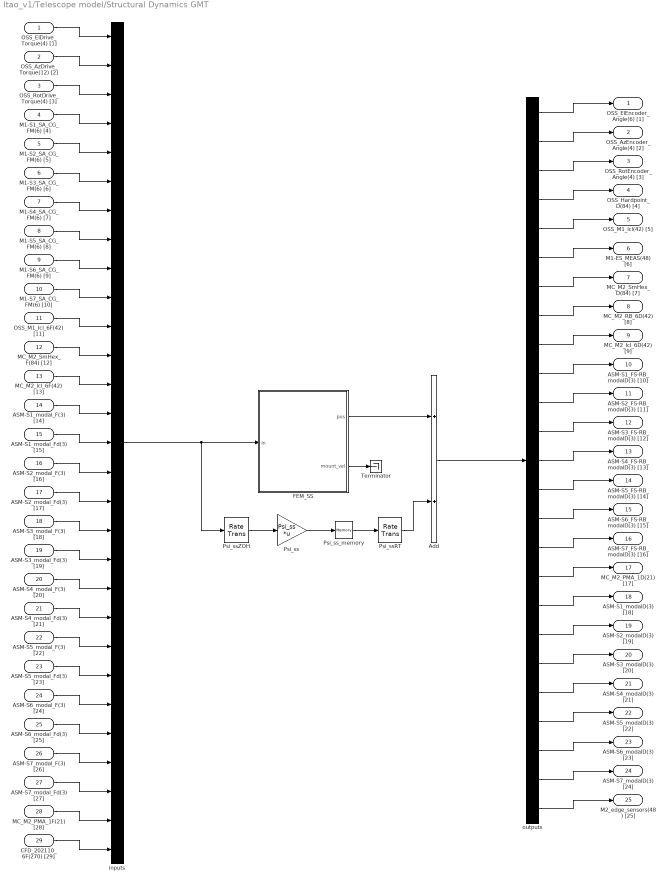
== system ltao_v1/Telescope model/Structural Dynamics GMT ==
  OSS_ElDrive_Torque(4) [1] : Inport  PortDimensions=4
  OSS_AzDrive_Torque(12) [2] : Inport  Port=2  PortDimensions=12
  OSS_RotDrive_Torque(4) [3] : Inport  Port=3  PortDimensions=4
  M1-S1_SA_CG_FM(6) [4] : Inport  Port=4  PortDimensions=6
  M1-S2_SA_CG_FM(6) [5] : Inport  Port=5  PortDimensions=6
  M1-S3_SA_CG_FM(6) [6] : Inport  Port=6  PortDimensions=6
  M1-S4_SA_CG_FM(6) [7] : Inport  Port=7  PortDimensions=6
  M1-S5_SA_CG_FM(6) [8] : Inport  Port=8  PortDimensions=6
  M1-S6_SA_CG_FM(6) [9] : Inport  Port=9  PortDimensions=6
  M1-S7_SA_CG_FM(6) [10] : Inport  Port=10  PortDimensions=6
  OSS_M1_lcl_6F(42) [11] : Inport  Port=11  PortDimensions=42
  MC_M2_SmHex_F(84) [12] : Inport  Port=12  PortDimensions=84
  MC_M2_lcl_6F(42) [13] : Inport  Port=13  PortDimensions=42
  ASM-S1_modal_F(3) [14] : Inport  Port=14  PortDimensions=3
  ASM-S1_modal_Fd(3) [15] : Inport  Port=15  PortDimensions=3
  ASM-S2_modal_F(3) [16] : Inport  Port=16  PortDimensions=3
  ASM-S2_modal_Fd(3) [17] : Inport  Port=17  PortDimensions=3
  ASM-S3_modal_F(3) [18] : Inport  Port=18  PortDimensions=3
  ASM-S3_modal_Fd(3) [19] : Inport  Port=19  PortDimensions=3
  ASM-S4_modal_F(3) [20] : Inport  Port=20  PortDimensions=3
  ASM-S4_modal_Fd(3) [21] : Inport  Port=21  PortDimensions=3
  ASM-S5_modal_F(3) [22] : Inport  Port=22  PortDimensions=3
  ASM-S5_modal_Fd(3) [23] : Inport  Port=23  PortDimensions=3
  ASM-S6_modal_F(3) [24] : Inport  Port=24  PortDimensions=3
  ASM-S6_modal_Fd(3) [25] : Inport  Port=25  PortDimensions=3
  ASM-S7_modal_F(3) [26] : Inport  Port=26  PortDimensions=3
  ASM-S7_modal_Fd(3) [27] : Inport  Port=27  PortDimensions=3
  MC_M2_PMA_1F(21) [28] : Inport  Port=28  PortDimensions=21
  CFD_202110_6F(270) [29] : Inport  Port=29  PortDimensions=270
  Add : Sum
  FEM_SS : Subsystem
  Psi_ss : Gain  Gain=Psi_ss  Multiplication=Matrix(K*u) (u vector)
  Psi_ssRT : RateTransition  Integrity=off  OutPortSampleTimeOpt=Inherit
  Psi_ssZOH : RateTransition  Integrity=off  OutPortSampleTime=Psi_ssTs
  Psi_ss_memory : Memory  InitialCondition=zeros(size(phiC,1),1)  InheritSampleTime=on  LinearizeAsDelay=on
  Terminator : Terminator
  inputs : Mux  Inputs=modelMuxDims
  outputs : Demux  Outputs=modelDemuxDims
  OSS_ElEncoder_Angle(6) [1] : Outport  PortDimensions=6
  OSS_AzEncoder_Angle(4) [2] : Outport  Port=2  PortDimensions=4
  OSS_RotEncoder_Angle(4) [3] : Outport  Port=3  PortDimensions=4
  OSS_Hardpoint_D(84) [4] : Outport  Port=4  PortDimensions=84
  OSS_M1_lcl(42) [5] : Outport  Port=5  PortDimensions=42
  M1-ES_MEAS(48) [6] : Outport  Port=6  PortDimensions=48
  MC_M2_SmHex_D(84) [7] : Outport  Port=7  PortDimensions=84
  MC_M2_RB_6D(42) [8] : Outport  Port=8  PortDimensions=42
  MC_M2_lcl_6D(42) [9] : Outport  Port=9  PortDimensions=42
  ASM-S1_FS-RB_modalD(3) [10] : Outport  Port=10  PortDimensions=3
  ASM-S2_FS-RB_modalD(3) [11] : Outport  Port=11  PortDimensions=3
  ASM-S3_FS-RB_modalD(3) [12] : Outport  Port=12  PortDimensions=3
  ASM-S4_FS-RB_modalD(3) [13] : Outport  Port=13  PortDimensions=3
  ASM-S5_FS-RB_modalD(3) [14] : Outport  Port=14  PortDimensions=3
  ASM-S6_FS-RB_modalD(3) [15] : Outport  Port=15  PortDimensions=3
  ASM-S7_FS-RB_modalD(3) [16] : Outport  Port=16  PortDimensions=3
  MC_M2_PMA_1D(21) [17] : Outport  Port=17  PortDimensions=21
  ASM-S1_modalD(3) [18] : Outport  Port=18  PortDimensions=3
  ASM-S2_modalD(3) [19] : Outport  Port=19  PortDimensions=3
  ASM-S3_modalD(3) [20] : Outport  Port=20  PortDimensions=3
  ASM-S4_modalD(3) [21] : Outport  Port=21  PortDimensions=3
  ASM-S5_modalD(3) [22] : Outport  Port=22  PortDimensions=3
  ASM-S6_modalD(3) [23] : Outport  Port=23  PortDimensions=3
  ASM-S7_modalD(3) [24] : Outport  Port=24  PortDimensions=3
  M2_edge_sensors(48) [25] : Outport  Port=25  PortDimensions=48
  wires:
  Add/1 -> outputs/1
  Psi_ssZOH/1 -> Psi_ss/1
  FEM_SS/2(mount_vel) -> Terminator/1
  FEM_SS/1(pos) -> Add/1
  inputs/1 -> FEM_SS/1(In), Psi_ssZOH/1
  Psi_ssRT/1 -> Add/2
  Psi_ss/1 -> Psi_ss_memory/1
  Psi_ss_memory/1 -> Psi_ssRT/1
  outputs/25 -> M2_edge_sensors(48) [25]/1
  outputs/24 -> ASM-S7_modalD(3) [24]/1
  outputs/23 -> ASM-S6_modalD(3) [23]/1
  outputs/22 -> ASM-S5_modalD(3) [22]/1
  outputs/21 -> ASM-S4_modalD(3) [21]/1
  outputs/20 -> ASM-S3_modalD(3) [20]/1
  outputs/19 -> ASM-S2_modalD(3) [19]/1
  outputs/18 -> ASM-S1_modalD(3) [18]/1
  outputs/17 -> MC_M2_PMA_1D(21) [17]/1
  outputs/16 -> ASM-S7_FS-RB_modalD(3) [16]/1
  outputs/15 -> ASM-S6_FS-RB_modalD(3) [15]/1
  outputs/14 -> ASM-S5_FS-RB_modalD(3) [14]/1
  outputs/13 -> ASM-S4_FS-RB_modalD(3) [13]/1
  outputs/12 -> ASM-S3_FS-RB_modalD(3) [12]/1
  outputs/11 -> ASM-S2_FS-RB_modalD(3) [11]/1
  outputs/10 -> ASM-S1_FS-RB_modalD(3) [10]/1
  outputs/9 -> MC_M2_lcl_6D(42) [9]/1
  outputs/8 -> MC_M2_RB_6D(42) [8]/1
  outputs/7 -> MC_M2_SmHex_D(84) [7]/1
  outputs/6 -> M1-ES_MEAS(48) [6]/1
  outputs/5 -> OSS_M1_lcl(42) [5]/1
  outputs/4 -> OSS_Hardpoint_D(84) [4]/1
  outputs/3 -> OSS_RotEncoder_Angle(4) [3]/1
  outputs/2 -> OSS_AzEncoder_Angle(4) [2]/1
  outputs/1 -> OSS_ElEncoder_Angle(6) [1]/1
  CFD_202110_6F(270) [29]/1 -> inputs/29
  MC_M2_PMA_1F(21) [28]/1 -> inputs/28
  ASM-S7_modal_Fd(3) [27]/1 -> inputs/27
  ASM-S7_modal_F(3) [26]/1 -> inputs/26
  ASM-S6_modal_Fd(3) [25]/1 -> inputs/25
  ASM-S6_modal_F(3) [24]/1 -> inputs/24
  ASM-S5_modal_Fd(3) [23]/1 -> inputs/23
  ASM-S5_modal_F(3) [22]/1 -> inputs/22
  ASM-S4_modal_Fd(3) [21]/1 -> inputs/21
  ASM-S4_modal_F(3) [20]/1 -> inputs/20
  ASM-S3_modal_Fd(3) [19]/1 -> inputs/19
  ASM-S3_modal_F(3) [18]/1 -> inputs/18
  ASM-S2_modal_Fd(3) [17]/1 -> inputs/17
  ASM-S2_modal_F(3) [16]/1 -> inputs/16
  ASM-S1_modal_Fd(3) [15]/1 -> inputs/15
  ASM-S1_modal_F(3) [14]/1 -> inputs/14
  MC_M2_lcl_6F(42) [13]/1 -> inputs/13
  MC_M2_SmHex_F(84) [12]/1 -> inputs/12
  OSS_M1_lcl_6F(42) [11]/1 -> inputs/11
  M1-S7_SA_CG_FM(6) [10]/1 -> inputs/10
  M1-S6_SA_CG_FM(6) [9]/1 -> inputs/9
  M1-S5_SA_CG_FM(6) [8]/1 -> inputs/8
  M1-S4_SA_CG_FM(6) [7]/1 -> inputs/7
  M1-S3_SA_CG_FM(6) [6]/1 -> inputs/6
  M1-S2_SA_CG_FM(6) [5]/1 -> inputs/5
  M1-S1_SA_CG_FM(6) [4]/1 -> inputs/4
  OSS_RotDrive_Torque(4) [3]/1 -> inputs/3
  OSS_AzDrive_Torque(12) [2]/1 -> inputs/2
  OSS_ElDrive_Torque(4) [1]/1 -> inputs/1

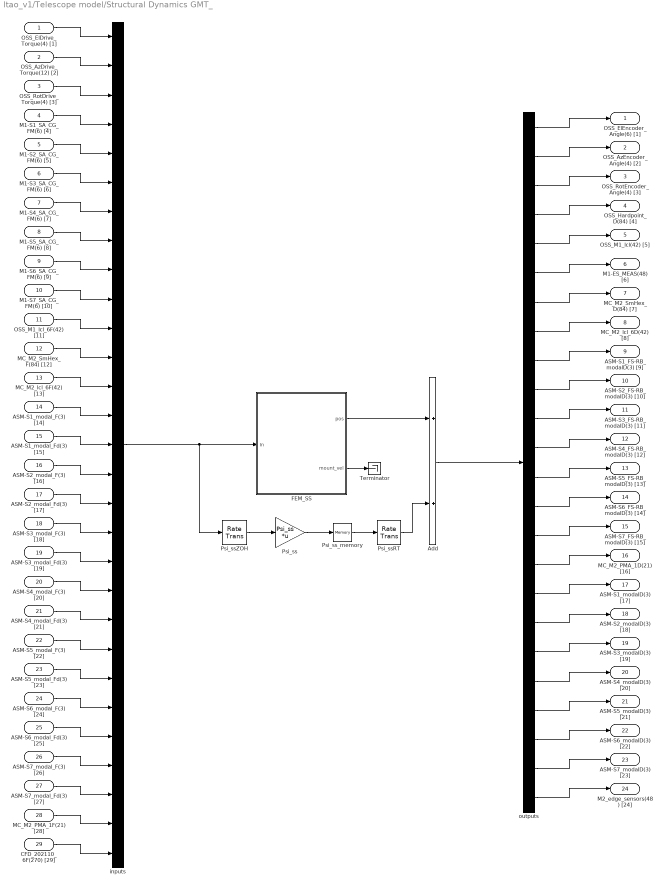
== system ltao_v1/Telescope model/Structural Dynamics GMT_ ==
  OSS_ElDrive_Torque(4) [1] : Inport  PortDimensions=4
  OSS_AzDrive_Torque(12) [2] : Inport  Port=2  PortDimensions=12
  OSS_RotDrive_Torque(4) [3] : Inport  Port=3  PortDimensions=4
  M1-S1_SA_CG_FM(6) [4] : Inport  Port=4  PortDimensions=6
  M1-S2_SA_CG_FM(6) [5] : Inport  Port=5  PortDimensions=6
  M1-S3_SA_CG_FM(6) [6] : Inport  Port=6  PortDimensions=6
  M1-S4_SA_CG_FM(6) [7] : Inport  Port=7  PortDimensions=6
  M1-S5_SA_CG_FM(6) [8] : Inport  Port=8  PortDimensions=6
  M1-S6_SA_CG_FM(6) [9] : Inport  Port=9  PortDimensions=6
  M1-S7_SA_CG_FM(6) [10] : Inport  Port=10  PortDimensions=6
  OSS_M1_lcl_6F(42) [11] : Inport  Port=11  PortDimensions=42
  MC_M2_SmHex_F(84) [12] : Inport  Port=12  PortDimensions=84
  MC_M2_lcl_6F(42) [13] : Inport  Port=13  PortDimensions=42
  ASM-S1_modal_F(3) [14] : Inport  Port=14  PortDimensions=3
  ASM-S1_modal_Fd(3) [15] : Inport  Port=15  PortDimensions=3
  ASM-S2_modal_F(3) [16] : Inport  Port=16  PortDimensions=3
  ASM-S2_modal_Fd(3) [17] : Inport  Port=17  PortDimensions=3
  ASM-S3_modal_F(3) [18] : Inport  Port=18  PortDimensions=3
  ASM-S3_modal_Fd(3) [19] : Inport  Port=19  PortDimensions=3
  ASM-S4_modal_F(3) [20] : Inport  Port=20  PortDimensions=3
  ASM-S4_modal_Fd(3) [21] : Inport  Port=21  PortDimensions=3
  ASM-S5_modal_F(3) [22] : Inport  Port=22  PortDimensions=3
  ASM-S5_modal_Fd(3) [23] : Inport  Port=23  PortDimensions=3
  ASM-S6_modal_F(3) [24] : Inport  Port=24  PortDimensions=3
  ASM-S6_modal_Fd(3) [25] : Inport  Port=25  PortDimensions=3
  ASM-S7_modal_F(3) [26] : Inport  Port=26  PortDimensions=3
  ASM-S7_modal_Fd(3) [27] : Inport  Port=27  PortDimensions=3
  MC_M2_PMA_1F(21) [28] : Inport  Port=28  PortDimensions=21
  CFD_202110_6F(270) [29] : Inport  Port=29  PortDimensions=270
  Add : Sum
  FEM_SS : Subsystem
  Psi_ss : Gain  Gain=Psi_ss  Multiplication=Matrix(K*u) (u vector)
  Psi_ssRT : RateTransition  Integrity=off  OutPortSampleTimeOpt=Inherit
  Psi_ssZOH : RateTransition  Integrity=off  OutPortSampleTime=Psi_ssTs
  Psi_ss_memory : Memory  InitialCondition=zeros(size(phiC,1),1)  InheritSampleTime=on  LinearizeAsDelay=on
  Terminator : Terminator
  inputs : Mux  Inputs=modelMuxDims
  outputs : Demux  Outputs=modelDemuxDims
  OSS_ElEncoder_Angle(6) [1] : Outport  PortDimensions=6
  OSS_AzEncoder_Angle(4) [2] : Outport  Port=2  PortDimensions=4
  OSS_RotEncoder_Angle(4) [3] : Outport  Port=3  PortDimensions=4
  OSS_Hardpoint_D(84) [4] : Outport  Port=4  PortDimensions=84
  OSS_M1_lcl(42) [5] : Outport  Port=5  PortDimensions=42
  M1-ES_MEAS(48) [6] : Outport  Port=6  PortDimensions=48
  MC_M2_SmHex_D(84) [7] : Outport  Port=7  PortDimensions=84
  MC_M2_lcl_6D(42) [8] : Outport  Port=8  PortDimensions=42
  ASM-S1_FS-RB_modalD(3) [9] : Outport  Port=9  PortDimensions=3
  ASM-S2_FS-RB_modalD(3) [10] : Outport  Port=10  PortDimensions=3
  ASM-S3_FS-RB_modalD(3) [11] : Outport  Port=11  PortDimensions=3
  ASM-S4_FS-RB_modalD(3) [12] : Outport  Port=12  PortDimensions=3
  ASM-S5_FS-RB_modalD(3) [13] : Outport  Port=13  PortDimensions=3
  ASM-S6_FS-RB_modalD(3) [14] : Outport  Port=14  PortDimensions=3
  ASM-S7_FS-RB_modalD(3) [15] : Outport  Port=15  PortDimensions=3
  MC_M2_PMA_1D(21) [16] : Outport  Port=16  PortDimensions=21
  ASM-S1_modalD(3) [17] : Outport  Port=17  PortDimensions=3
  ASM-S2_modalD(3) [18] : Outport  Port=18  PortDimensions=3
  ASM-S3_modalD(3) [19] : Outport  Port=19  PortDimensions=3
  ASM-S4_modalD(3) [20] : Outport  Port=20  PortDimensions=3
  ASM-S5_modalD(3) [21] : Outport  Port=21  PortDimensions=3
  ASM-S6_modalD(3) [22] : Outport  Port=22  PortDimensions=3
  ASM-S7_modalD(3) [23] : Outport  Port=23  PortDimensions=3
  M2_edge_sensors(48) [24] : Outport  Port=24  PortDimensions=48
  wires:
  outputs/24 -> M2_edge_sensors(48) [24]/1
  outputs/23 -> ASM-S7_modalD(3) [23]/1
  outputs/22 -> ASM-S6_modalD(3) [22]/1
  outputs/21 -> ASM-S5_modalD(3) [21]/1
  outputs/20 -> ASM-S4_modalD(3) [20]/1
  outputs/19 -> ASM-S3_modalD(3) [19]/1
  outputs/18 -> ASM-S2_modalD(3) [18]/1
  outputs/17 -> ASM-S1_modalD(3) [17]/1
  outputs/16 -> MC_M2_PMA_1D(21) [16]/1
  outputs/15 -> ASM-S7_FS-RB_modalD(3) [15]/1
  outputs/14 -> ASM-S6_FS-RB_modalD(3) [14]/1
  outputs/13 -> ASM-S5_FS-RB_modalD(3) [13]/1
  outputs/12 -> ASM-S4_FS-RB_modalD(3) [12]/1
  outputs/11 -> ASM-S3_FS-RB_modalD(3) [11]/1
  outputs/10 -> ASM-S2_FS-RB_modalD(3) [10]/1
  outputs/9 -> ASM-S1_FS-RB_modalD(3) [9]/1
  outputs/8 -> MC_M2_lcl_6D(42) [8]/1
  outputs/7 -> MC_M2_SmHex_D(84) [7]/1
  outputs/6 -> M1-ES_MEAS(48) [6]/1
  outputs/5 -> OSS_M1_lcl(42) [5]/1
  outputs/4 -> OSS_Hardpoint_D(84) [4]/1
  outputs/3 -> OSS_RotEncoder_Angle(4) [3]/1
  outputs/2 -> OSS_AzEncoder_Angle(4) [2]/1
  outputs/1 -> OSS_ElEncoder_Angle(6) [1]/1
  Add/1 -> outputs/1
  CFD_202110_6F(270) [29]/1 -> inputs/29
  MC_M2_PMA_1F(21) [28]/1 -> inputs/28
  ASM-S7_modal_Fd(3) [27]/1 -> inputs/27
  ASM-S7_modal_F(3) [26]/1 -> inputs/26
  ASM-S6_modal_Fd(3) [25]/1 -> inputs/25
  ASM-S6_modal_F(3) [24]/1 -> inputs/24
  ASM-S5_modal_Fd(3) [23]/1 -> inputs/23
  ASM-S5_modal_F(3) [22]/1 -> inputs/22
  ASM-S4_modal_Fd(3) [21]/1 -> inputs/21
  ASM-S4_modal_F(3) [20]/1 -> inputs/20
  ASM-S3_modal_Fd(3) [19]/1 -> inputs/19
  ASM-S3_modal_F(3) [18]/1 -> inputs/18
  ASM-S2_modal_Fd(3) [17]/1 -> inputs/17
  ASM-S2_modal_F(3) [16]/1 -> inputs/16
  ASM-S1_modal_Fd(3) [15]/1 -> inputs/15
  ASM-S1_modal_F(3) [14]/1 -> inputs/14
  MC_M2_lcl_6F(42) [13]/1 -> inputs/13
  MC_M2_SmHex_F(84) [12]/1 -> inputs/12
  OSS_M1_lcl_6F(42) [11]/1 -> inputs/11
  M1-S7_SA_CG_FM(6) [10]/1 -> inputs/10
  M1-S6_SA_CG_FM(6) [9]/1 -> inputs/9
  M1-S5_SA_CG_FM(6) [8]/1 -> inputs/8
  M1-S4_SA_CG_FM(6) [7]/1 -> inputs/7
  M1-S3_SA_CG_FM(6) [6]/1 -> inputs/6
  M1-S2_SA_CG_FM(6) [5]/1 -> inputs/5
  M1-S1_SA_CG_FM(6) [4]/1 -> inputs/4
  OSS_RotDrive_Torque(4) [3]/1 -> inputs/3
  OSS_AzDrive_Torque(12) [2]/1 -> inputs/2
  OSS_ElDrive_Torque(4) [1]/1 -> inputs/1
  Psi_ss/1 -> Psi_ss_memory/1
  Psi_ssZOH/1 -> Psi_ss/1
  Psi_ss_memory/1 -> Psi_ssRT/1
  inputs/1 -> Psi_ssZOH/1, FEM_SS/1(In)
  FEM_SS/1(pos) -> Add/1
  FEM_SS/2(mount_vel) -> Terminator/1
  Psi_ssRT/1 -> Add/2

== system ltao_v1/Wind Loads/Sigmoid ==
  Add : Sum  Inputs=+-
  Add1 : Sum
  Clock : Clock
  Constant : Constant  Value=0.75
  CteOne : Constant
  Gain : Gain  Gain=-5
  Math Function : Math  SignedPower=on
  Reciprocal Function : Math  Operator=reciprocal  SignedPower=on
  Sqr Function : Math  Operator=square  SignedPower=on
  s : Outport
  wires:
  Sqr Function/1 -> Reciprocal Function/1
  Math Function/1 -> Add1/2
  Gain/1 -> Math Function/1
  Add/1 -> Gain/1
  Clock/1 -> Add/1
  Constant/1 -> Add/2
  Add1/1 -> Sqr Function/1
  CteOne/1 -> Add1/1
  Reciprocal Function/1 -> s/1

== system ltao_v1/gTT Controller/segPTT2asmCMD ==
  segTTP : Inport
  Mux : Mux  Inputs=7
  PTT2ASM_S1 : Gain  Gain=segPTT2asmCMD{1}  Multiplication=Matrix(K*u)
  PTT2ASM_S2 : Gain  Gain=segPTT2asmCMD{2}  Multiplication=Matrix(K*u)
  PTT2ASM_S3 : Gain  Gain=segPTT2asmCMD{3}  Multiplication=Matrix(K*u)
  PTT2ASM_S4 : Gain  Gain=segPTT2asmCMD{4}  Multiplication=Matrix(K*u)
  PTT2ASM_S5 : Gain  Gain=segPTT2asmCMD{5}  Multiplication=Matrix(K*u)
  PTT2ASM_S6 : Gain  Gain=segPTT2asmCMD{6}  Multiplication=Matrix(K*u)
  PTT2ASM_S7 : Gain  Gain=segPTT2asmCMD{7}  Multiplication=Matrix(K*u)
  Selector_S1 : Selector  InputPortWidth=21  IndexOptions=Index vector (dialog)  Indices=1:7:21  OutputSizes=1
  Selector_S2 : Selector  InputPortWidth=21  IndexOptions=Index vector (dialog)  Indices=2:7:21  OutputSizes=1
  Selector_S3 : Selector  InputPortWidth=21  IndexOptions=Index vector (dialog)  Indices=3:7:21  OutputSizes=1
  Selector_S4 : Selector  InputPortWidth=21  IndexOptions=Index vector (dialog)  Indices=4:7:21  OutputSizes=1
  Selector_S5 : Selector  InputPortWidth=21  IndexOptions=Index vector (dialog)  Indices=5:7:21  OutputSizes=1
  Selector_S6 : Selector  InputPortWidth=21  IndexOptions=Index vector (dialog)  Indices=6:7:21  OutputSizes=1
  Selector_S7 : Selector  InputPortWidth=21  IndexOptions=Index vector (dialog)  Indices=7:7:21  OutputSizes=1
  ASM_KL012_CMD : Outport
  wires:
  Mux/1 -> ASM_KL012_CMD/1
  PTT2ASM_S7/1 -> Mux/7
  PTT2ASM_S6/1 -> Mux/6
  PTT2ASM_S5/1 -> Mux/5
  PTT2ASM_S3/1 -> Mux/3
  PTT2ASM_S4/1 -> Mux/4
  PTT2ASM_S2/1 -> Mux/2
  Selector_S4/1 -> PTT2ASM_S4/1
  PTT2ASM_S1/1 -> Mux/1
  Selector_S7/1 -> PTT2ASM_S7/1
  Selector_S6/1 -> PTT2ASM_S6/1
  Selector_S3/1 -> PTT2ASM_S3/1
  Selector_S2/1 -> PTT2ASM_S2/1
  Selector_S1/1 -> PTT2ASM_S1/1
  Selector_S5/1 -> PTT2ASM_S5/1
  segTTP/1 -> Selector_S7/1, Selector_S6/1, Selector_S5/1, Selector_S4/1, Selector_S3/1, Selector_S2/1, Selector_S1/1

== system ltao_v1/ASMmodal_Control/ASM_inner_loop_controller_S2/Pre shape + FF terms ==
  cmd : Inport  PortDimensions=length(VC_modal_stiff{1})
  " 1" : Constant  Commented=on  Value=sm.tSF
  " 2" : Constant  Commented=on  Value=sm.d1SF
  " 3" : Constant  Commented=on  Value=sm.d2SF
  " 4" : Constant  Commented=on  Value=sm.d3SF
  " 5" : Constant  Commented=on  Value=sm.TCmd
  Clock : Clock  Commented=on
  Cmd Shaping Filter : Subsystem
  Command Shaping Filter : MATLAB Function  Commented=on  TreatAsAtomicUnit=on  SystemSampleTime=FEM_Ts
  Memory : Memory  Commented=on  InheritSampleTime=on
  Mux : Mux  Commented=on  Inputs=2
  RTout : RateTransition  Commented=on  OutPortSampleTime=FEM_Ts
  RTout_CMdOld : RateTransition  Commented=on  OutPortSampleTime=FEM_Ts
  Scope : Scope  Commented=on
  Selector : Selector  Commented=on  InputPortWidth=66  IndexOptions=Index vector (dialog)  Indices=[1 2 4]  OutputSizes=1
  Selector1 : Selector  Commented=on  InputPortWidth=66  IndexOptions=Index vector (dialog)  Indices=[1 2 4]  OutputSizes=1
  SFdd : Outport  PortDimensions=length(VC_modal_stiff{1})  VectorParamsAs1DForOutWhenUnconnected=off
  SFd : Outport  Port=2  PortDimensions=length(VC_modal_stiff{1})  VectorParamsAs1DForOutWhenUnconnected=off
  SF : Outport  Port=3  PortDimensions=length(VC_modal_stiff{1})  VectorParamsAs1DForOutWhenUnconnected=off
  wires:
  " 4"/1 -> Command Shaping Filter/8(d3SF)
  Clock/1 -> Command Shaping Filter/3(t)
  cmd/1 -> RTout/1, Memory/1, Cmd Shaping Filter/1(cmd)
  " 1"/1 -> Command Shaping Filter/5(tSF)
  " 3"/1 -> Command Shaping Filter/7(d2SF)
  " 2"/1 -> Command Shaping Filter/6(d1SF)
  Memory/1 -> RTout_CMdOld/1
  RTout/1 -> Command Shaping Filter/2(cmd)
  RTout_CMdOld/1 -> Command Shaping Filter/1(cmdOld)
  Selector/1 -> Mux/1
  Selector1/1 -> Mux/2
  Mux/1 -> Scope/1
  " 5"/1 -> Command Shaping Filter/4(Tcmd)
  Cmd Shaping Filter/3(SF) -> SF/1
  Cmd Shaping Filter/1(SFdd) -> SFdd/1, Selector/1
  Cmd Shaping Filter/2(SFd) -> SFd/1
  Command Shaping Filter/1(cmdSFdd) -> Selector1/1

== system ltao_v1/Mount_Drv_PDR2021_linear/AZ DT Lugre Fr model/g(v) ==
  v : Inport
  Enable : EnablePort
  Constant : Constant  Value=0
  gs : Subsystem
  g : Outport  VectorParamsAs1DForOutWhenUnconnected=off
  wires:
  gs/1(gs(v)) -> g/1
  v/1 -> gs/1(v)
  Constant/1 -> gs/Enable

== system ltao_v1/Mount_Drv_PDR2021_linear/AZ DT Lugre Fr model/v2z ==
  v : Inport
  g(v) : Inport  Port=2
  z : Inport  Port=3
  Enable : EnablePort
  Abs : Abs  SaturateOnIntegerOverflow=off
  Divide : Product  Inputs=*/*
  Sum : Sum  Inputs=|+-
  dz : Outport  VectorParamsAs1DForOutWhenUnconnected=off
  wires:
  Abs/1 -> Divide/1
  Divide/1 -> Sum/2
  v/1 -> Sum/1, Abs/1
  Sum/1 -> dz/1
  g(v)/1 -> Divide/2
  z/1 -> Divide/3

== system ltao_v1/Mount_Drv_PDR2021_linear/EL DT Lugre Fr model/g(v) ==
  v : Inport
  Enable : EnablePort
  Constant : Constant  Value=0
  Sum : Sum  Inputs=|++
  gc : Constant  Value=frParStruct.Tc/frParStruct.sigm0
  gs : Subsystem
  g : Outport  VectorParamsAs1DForOutWhenUnconnected=off
  wires:
  Sum/1 -> g/1
  v/1 -> gs/1(v)
  gs/1(gs(v)) -> Sum/1
  gc/1 -> Sum/2
  Constant/1 -> gs/Enable

== system ltao_v1/Mount_Drv_PDR2021_linear/EL DT Lugre Fr model/v2z ==
  v : Inport
  g(v) : Inport  Port=2
  z : Inport  Port=3
  Enable : EnablePort
  Abs : Abs  SaturateOnIntegerOverflow=off
  Divide : Product  Inputs=*/*
  Sum : Sum  Inputs=|+-
  dz : Outport  VectorParamsAs1DForOutWhenUnconnected=off
  wires:
  Abs/1 -> Divide/1
  Divide/1 -> Sum/2
  v/1 -> Sum/1, Abs/1
  Sum/1 -> dz/1
  g(v)/1 -> Divide/2
  z/1 -> Divide/3

== system ltao_v1/Mount_Drv_PDR2021_linear/GIR DT Lugre Fr model/g(v) ==
  v : Inport
  Constant : Constant  Value=0
  Sum : Sum  Inputs=|++
  gc : Constant  Value=frParStruct.Tc/frParStruct.sigm0
  gs : Subsystem
  g : Outport  VectorParamsAs1DForOutWhenUnconnected=off
  wires:
  Sum/1 -> g/1
  v/1 -> gs/1(v)
  gs/1(gs(v)) -> Sum/1
  gc/1 -> Sum/2
  Constant/1 -> gs/Enable
